simulink model "manipTransformTrajectoryTimeScaling"  (R2021a)
settings: Solver=FixedStepAuto  StartTime=0.0  StopTime=inf  RelTol=1e-3
PreLoadFcn:
  | createWaypointData;
undefined symbols (not defined in the file): eul2tform, gen3, maxWaypoints, trvec2tform, ts
libraries: trajExampleUtils x6, robotcorelib x3, robotmaniplib x1
settings Model: Creator=scastro  LastModifiedBy=dzy
settings SolverCC: AlgebraicLoopSolver=TrustRegion
settings DataIOCC: ReturnWorkspaceOutputs=off
settings OptimizationCC: DefaultParameterBehavior=Inlined  EnhancedBackFolding=on  PassReuseOutputArgsAs=Individual arguments  OptimizeBlockOrder=speed  DifferentSizesBufferReuse=on  OptimizationCustomize=off  EfficientTunableParamExpr=on
settings DebuggingCC: ParameterTunabilityLossMsg=error  SFMachineParentedDataDiag=warning  ArithmeticOperatorsInVariantConditions=warning
settings SFSimCC: CustomCodeUndefinedFunction=UseInterfaceOnly
settings RTWCC: SystemTargetFile=ert.tlc  TemplateMakefile=ert_default_tmf  GenerateReport=on  IncludeHyperlinkInReport=on  LaunchReport=on  GenerateTraceInfo=on  GenerateTraceReport=on  GenerateTraceReportSl=on  GenerateTraceReportSf=on  GenerateTraceReportEml=on
settings CodeAppCC: ForceParamTrailComments=on  IgnoreCustomStorageClasses=off  OperatorAnnotations=on  SimulinkDataObjDesc=on  SFDataObjDesc=on  InsertBlockDesc=on
settings ERTTargetCC: TargetLangStandard=C99 (ISO)  GenerateSampleERTMain=on  SupportVariableSizeSignals=on  InlinedParameterPlacement=NonHierarchical  ERTCustomFileTemplate=example_file_process.tlc

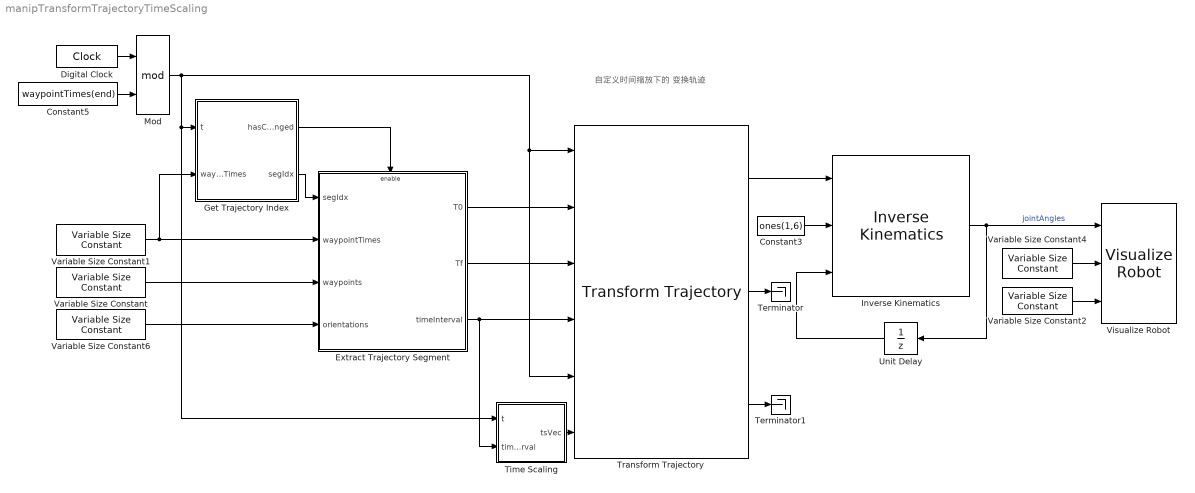
== system manipTransformTrajectoryTimeScaling ==
  note: 自定义时间缩放下的 变换轨迹
  Constant3 : Constant  Value=ones(1,6)  VectorParams1D=off
  Constant5 : Constant  Value=waypointTimes(end)
  Digital Clock : DigitalClock  SampleTime=ts
  Extract Trajectory Segment : Subsystem
  Get Trajectory Index : MATLAB Function  TreatAsAtomicUnit=on
  Inverse Kinematics : robotmaniplib/Inverse Kinematics  RigidBodyTree=gen3  EndEffector=Gripper  ShowInfo=off  SolverName=BFGS Gradient Projection  EnforceJointLimits=on  MaxIterations=1500  MaxTime=10  GradientTolerance=1e-7  SolutionTolerance=1e-6  StepTolerance=1e-14  ErrorChangeTolerance=1e-12  UseErrorDamping=on  DampingBias=0.0025  SimulateUsing=Interpreted execution
  Mod : Math  Operator=mod  SignedPower=on  SaturateOnIntegerOverflow=on
  Terminator : Terminator
  Terminator1 : Terminator
  Time Scaling : Subsystem
  Transform Trajectory : robotcorelib/Transform Trajectory  WaypointSource=External  T0=trvec2tform( [ 1, 10, -1 ] )  TF=eul2tform( [ 0, pi, pi / 2 ] )  TimeInterval=[ 2, 3 ]  CustomTimeScaling=on  ParameterSource=External  TSTime=2:0.1:3  TimeScaling=[ 0:0.1:1; ones( 1, 11 ); zeros( 1, 11 ) ]  SimulateUsing=Interpreted execution
      settings: SourceProductBaseCode=NV,RO,RR,UV
  Unit Delay : UnitDelay  InitialCondition=ikInitGuess'  SampleTime=-1  HasFrameUpgradeWarning=on
  Variable Size Constant : trajExampleUtils/Variable Size Constant  val=waypoints  maxSize=[3,maxWaypoints]  Ts=-1
  Variable Size Constant1 : trajExampleUtils/Variable Size Constant  val=waypointTimes  maxSize=[1,maxWaypoints]  Ts=-1
  Variable Size Constant2 : trajExampleUtils/Variable Size Constant  val=orientations  maxSize=[3,maxWaypoints]  Ts=-1
  Variable Size Constant4 : trajExampleUtils/Variable Size Constant  val=waypoints  maxSize=[3,maxWaypoints]  Ts=-1
  Variable Size Constant6 : trajExampleUtils/Variable Size Constant  val=orientations  maxSize=[3,maxWaypoints]  Ts=-1
  Visualize Robot : trajExampleUtils/Visualize Robot  rbtName=gen3  eeName=Gripper  numJoints=numel(gen3.homeConfiguration)  maxPts=maxWaypoints  plotMode=Coordinate Frames
  wires:
  Digital Clock/1 -> Mod/1
  Variable Size Constant1/1 -> Extract Trajectory Segment/2(waypointTimes), Get Trajectory Index/2(waypointTimes)
  Transform Trajectory/1 -> Inverse Kinematics/1
  Constant3/1 -> Inverse Kinematics/2
  Inverse Kinematics/1 -> Visualize Robot/1, Unit Delay/1  "jointAngles"
  Mod/1 -> Transform Trajectory/1, Transform Trajectory/5, Time Scaling/1(t), Get Trajectory Index/1(t)
  Constant5/1 -> Mod/2
  Unit Delay/1 -> Inverse Kinematics/3
  Variable Size Constant4/1 -> Visualize Robot/2
  Transform Trajectory/2 -> Terminator/1
  Transform Trajectory/3 -> Terminator1/1
  Get Trajectory Index/2(segIdx) -> Extract Trajectory Segment/1(segIdx)
  Variable Size Constant/1 -> Extract Trajectory Segment/3(waypoints)
  Variable Size Constant6/1 -> Extract Trajectory Segment/4(orientations)
  Extract Trajectory Segment/1(T0) -> Transform Trajectory/2
  Extract Trajectory Segment/2(Tf) -> Transform Trajectory/3
  Get Trajectory Index/1(hasChanged) -> Extract Trajectory Segment/Enable
  Extract Trajectory Segment/3(timeInterval) -> Transform Trajectory/4, Time Scaling/2(timeInterval)
  Time Scaling/1(tsVec) -> Transform Trajectory/6
  Variable Size Constant2/1 -> Visualize Robot/3

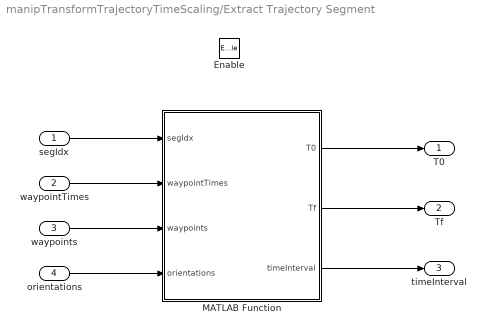
== system manipTransformTrajectoryTimeScaling/Extract Trajectory Segment ==
  segIdx : Inport
  waypointTimes : Inport  Port=2
  waypoints : Inport  Port=3
  orientations : Inport  Port=4
  Enable : EnablePort  PropagateVarSize=During execution
  MATLAB Function : MATLAB Function  TreatAsAtomicUnit=on
  T0 : Outport  VectorParamsAs1DForOutWhenUnconnected=off
  Tf : Outport  Port=2  VectorParamsAs1DForOutWhenUnconnected=off
  timeInterval : Outport  Port=3  VectorParamsAs1DForOutWhenUnconnected=off
  wires:
  segIdx/1 -> MATLAB Function/1(segIdx)
  MATLAB Function/1(T0) -> T0/1
  MATLAB Function/3(timeInterval) -> timeInterval/1
  orientations/1 -> MATLAB Function/4(orientations)
  waypoints/1 -> MATLAB Function/3(waypoints)
  MATLAB Function/2(Tf) -> Tf/1
  waypointTimes/1 -> MATLAB Function/2(waypointTimes)

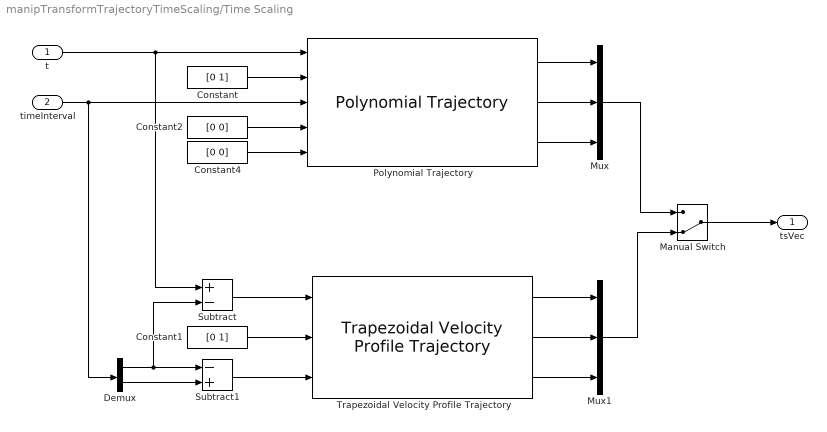
== system manipTransformTrajectoryTimeScaling/Time Scaling ==
  t : Inport
  timeInterval : Inport  Port=2
  Constant : Constant  Value=[0 1]  VectorParams1D=off
  Constant1 : Constant  Value=[0 1]  VectorParams1D=off
  Constant2 : Constant  Value=[0 0]  VectorParams1D=off
  Constant4 : Constant  Value=[0 0]  VectorParams1D=off
  Demux : Demux  Outputs=2
  Manual Switch : ManualSwitch  CurrentSetting=0
  Mux : Mux  Inputs=3
  Mux1 : Mux  Inputs=3
  Polynomial Trajectory : robotcorelib/Polynomial Trajectory  WaypointSource=External  Waypoints=[ 0, 2, 1, 5, 0; -1, 3, 1, 4, 4 ]  TimePoints=[ 0, 1, 2, 3, 4 ]  TimeInterval=[ 1, 4 ]  Method=Quintic Polynomial  ParameterSource=External  VelocityBoundaryCondition=zeros( 2, 5 )  AccelerationBoundaryCondition=zeros( 2, 5 )  SimulateUsing=Interpreted execution
  Subtract : Sum  Inputs=+-
  Subtract1 : Sum  Inputs=-+
  Trapezoidal Velocity Profile Trajectory : robotcorelib/Trapezoidal Velocity Profile Trajectory  WaypointSource=External  Waypoints=[ 0, -0.5, -1; 0, 0.5, 1 ]  NumParams=1  Parameter1=End Time  Parameter2=End Time  ParameterSource=External  PeakVelocity=[ 2; 2 ]  Acceleration=[ 1; 2 ]  EndTime=[ 1; 1 ]  AccelTime=[ 1; 2 ]  SimulateUsing=Interpreted execution
      settings: SourceProductBaseCode=NV,RO,RR,UV
  tsVec : Outport  VectorParamsAs1DForOutWhenUnconnected=off
  wires:
  Manual Switch/1 -> tsVec/1
  Polynomial Trajectory/3 -> Mux/3
  Polynomial Trajectory/1 -> Mux/1
  Constant/1 -> Polynomial Trajectory/2
  Constant4/1 -> Polynomial Trajectory/5
  Constant2/1 -> Polynomial Trajectory/4
  Polynomial Trajectory/2 -> Mux/2
  t/1 -> Polynomial Trajectory/1, Subtract/1
  Mux/1 -> Manual Switch/1
  Trapezoidal Velocity Profile Trajectory/1 -> Mux1/1
  Trapezoidal Velocity Profile Trajectory/2 -> Mux1/2
  Trapezoidal Velocity Profile Trajectory/3 -> Mux1/3
  Mux1/1 -> Manual Switch/2
  Constant1/1 -> Trapezoidal Velocity Profile Trajectory/2
  timeInterval/1 -> Demux/1, Polynomial Trajectory/3
  Subtract1/1 -> Trapezoidal Velocity Profile Trajectory/3
  Demux/1 -> Subtract/2, Subtract1/1
  Subtract/1 -> Trapezoidal Velocity Profile Trajectory/1
  Demux/2 -> Subtract1/2

== matlab function manipTransformTrajectoryTimeScaling/Get Trajectory Index ==
  data: hasChanged output; t input; segIdx output; waypointTimes input size=[1 maxWaypoints]
function [hasChanged,segIdx] = getTrajIdx(t,waypointTimes)

% Initialize previous index
persistent prevIdx
if isempty(prevIdx)
    prevIdx = 0;
end

% Find the trajectory segment index
segIndices = find(t>=waypointTimes);

% Limit the index value to the number of times minus one
% (This addresses the final time case)
segIdx = min(segIndices(end),numel(waypointTimes)-1);

% Determine whether the index has changed from the previous time step
if prevIdx == segIdx
    hasChanged = false;
else
    hasChanged = true;
    prevIdx = segIdx;
end

end

== matlab function manipTransformTrajectoryTimeScaling/Extract Trajectory Segment/MATLAB Function ==
  data: segIdx input; waypointTimes input size=[1 maxWaypoints]; T0 output size=[4 4]; waypoints input size=[3 maxWaypoints]; orientations input size=[3 maxWaypoints]; Tf output size=[4 4]; timeInterval output size=[1 2]
function [T0, Tf, timeInterval] = createTransformTrajSegment(segIdx,waypointTimes,waypoints,orientations)

% Extract the time interval, initial, and final transforms for the segment
timeInterval = waypointTimes(segIdx:segIdx+1);
T0 = trvec2tform(waypoints(:,segIdx)') * eul2tform(orientations(:,segIdx)');
Tf = trvec2tform(waypoints(:,segIdx+1)') * eul2tform(orientations(:,segIdx+1)');

end
